simulink model "modelo_bicicleta_backup"  (R2025a)
settings: Solver=VariableStepAuto  StartTime=0.0  StopTime=10.0  RelTol=1e-3
undefined symbols (not defined in the file): a, b, Caf, Car, Iz, m, vx
settings Model: Creator=Anderson  LastModifiedBy=Anderson

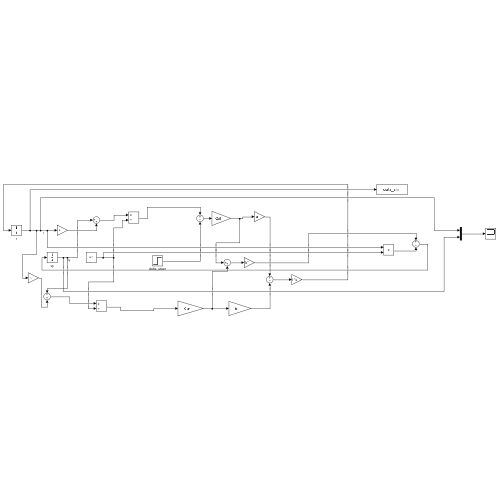
[thumbnail: Simulink's stored preview of the top-level diagram]
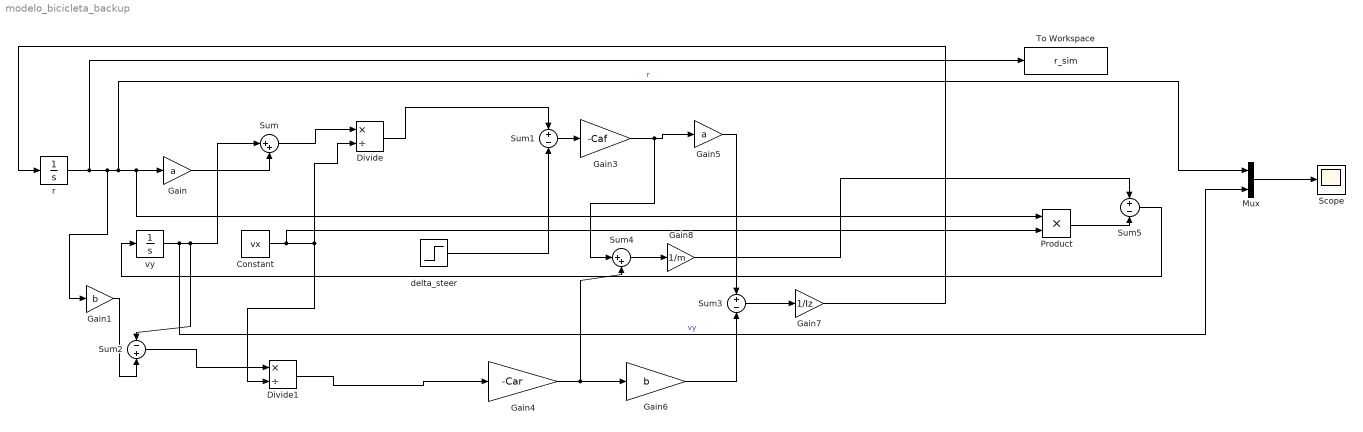
== system modelo_bicicleta_backup ==
  Constant : Constant  Value=vx
  Divide : Product  Inputs=*/
  Divide1 : Product  Inputs=*/
  Gain : Gain  Gain=a
  Gain1 : Gain  Gain=b
  Gain3 : Gain  Gain=-Caf
  Gain4 : Gain  Gain=-Car
  Gain5 : Gain  Gain=a
  Gain6 : Gain  Gain=b
  Gain7 : Gain  Gain=1/Iz
  Gain8 : Gain  Gain=1/m
  Mux : Mux  Inputs=2
  Product : Product
  Scope : Scope
      settings: Title=Resposta do Veículo a uma Entrada Degrau no Volante  ActiveDisplayYMinimum=-38.88920545293638  ActiveDisplayYMaximum=20.411145903131942
  Sum : Sum  Inputs=|++
  Sum1 : Sum  Inputs=+-
  Sum2 : Sum  Inputs=-+
  Sum3 : Sum  Inputs=+-
  Sum4 : Sum  Inputs=|++
  Sum5 : Sum  Inputs=+-
  To Workspace : ToWorkspace  VariableName=r_sim  SaveFormat=Timeseries  SampleTime=-1
  delta_steer : Step  After=0.1  SampleTime=0
  r : Integrator
  vy : Integrator
  wires:
  r/1 -> To Workspace/1, Gain1/1, Mux/1, Product/1, Gain/1  "r"
  vy/1 -> Mux/2, Sum/1, Sum2/1  "vy"
  Gain/1 -> Sum/2
  Sum/1 -> Divide/1
  Constant/1 -> Product/2, Divide/2, Divide1/2
  delta_steer/1 -> Sum1/2
  Divide/1 -> Sum1/1
  Gain1/1 -> Sum2/2
  Sum2/1 -> Divide1/1
  Sum1/1 -> Gain3/1
  Divide1/1 -> Gain4/1
  Gain4/1 -> Gain6/1, Sum4/2
  Gain3/1 -> Sum4/1, Gain5/1
  Gain5/1 -> Sum3/1
  Gain6/1 -> Sum3/2
  Sum3/1 -> Gain7/1
  Gain7/1 -> r/1
  Sum4/1 -> Gain8/1
  Gain8/1 -> Sum5/1
  Product/1 -> Sum5/2
  Sum5/1 -> vy/1
  Mux/1 -> Scope/1
